simulink model "WS1Sol"  (R2019b)
settings: Solver=VariableStepAuto  StartTime=0.0  StopTime=10  RelTol=1e-3
libraries: dspsrcs4 x2, simulink_extras x1
settings Model: Creator=Shishir  LastModifiedBy=Shishir

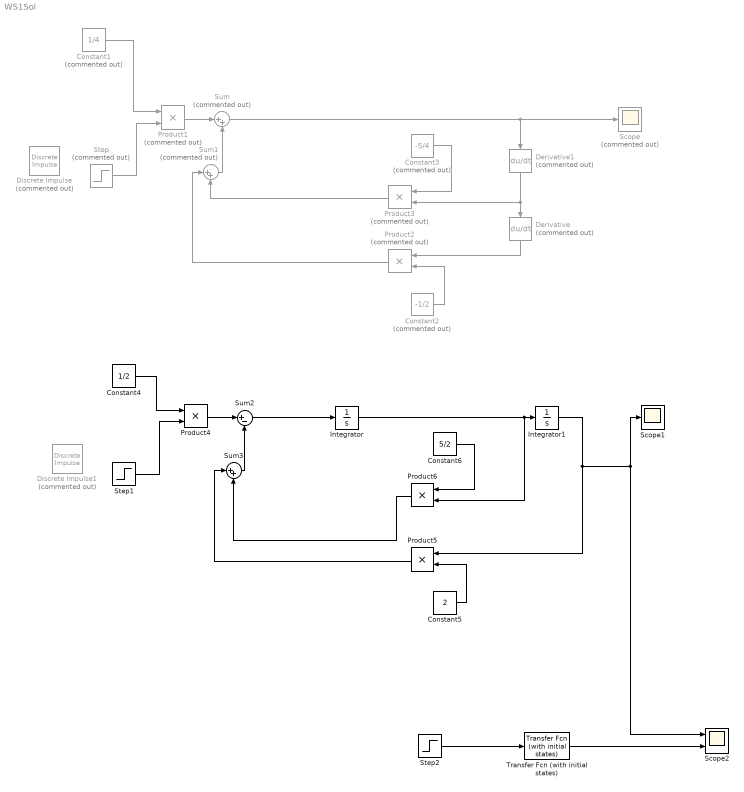
== system WS1Sol ==
  Constant1 : Constant  Commented=on  Value=1/4
  Constant2 : Constant  Commented=on  Value=-1/2
  Constant3 : Constant  Commented=on  Value=-5/4
  Constant4 : Constant  Value=1/2
  Constant5 : Constant  Value=2
  Constant6 : Constant  Value=5/2
  Derivative : Derivative  Commented=on
  Derivative1 : Derivative  Commented=on
  Discrete Impulse : dspsrcs4/Discrete  Impulse  Commented=on  Delay=0  SampleTime=1  FrameSample=1  OutputFrames=off  dataType=double  isSigned=on  wordLen=16  udDataType=sfix(16)  fracBitsMode=Best precision  numFracBits=15  OutDataTypeStr=double  LastOutDataTypeStr=double
  Discrete Impulse1 : dspsrcs4/Discrete  Impulse  Commented=on  Delay=0  SampleTime=1  FrameSample=1  OutputFrames=off  dataType=double  isSigned=on  wordLen=16  udDataType=sfix(16)  fracBitsMode=Best precision  numFracBits=15  OutDataTypeStr=double  LastOutDataTypeStr=double
  Integrator : Integrator
  Integrator1 : Integrator
  Product1 : Product  Commented=on
  Product2 : Product  Commented=on
  Product3 : Product  Commented=on
  Product4 : Product
  Product5 : Product
  Product6 : Product
  Scope : Scope  Commented=on
  Scope1 : Scope
  Scope2 : Scope  NumInputPorts=2
  Step : Step  Commented=on  SampleTime=0
  Step1 : Step  SampleTime=0
  Step2 : Step  SampleTime=0
  Sum : Sum  Commented=on  Inputs=|++
  Sum1 : Sum  Commented=on  Inputs=|++
  Sum2 : Sum  Inputs=|+-
  Sum3 : Sum  Inputs=|++
  Transfer Fcn (with initial states) : simulink_extras/Additional Linear/Transfer Fcn (with initial states)  N=[1]  D="[2  5 4]"  X0=0
  wires:
  Product1/1 -> Sum/1
  Step/1 -> Product1/2
  Constant1/1 -> Product1/1
  Sum/1 -> Derivative1/1, Scope/1
  Derivative1/1 -> Product3/2, Derivative/1
  Sum1/1 -> Sum/2
  Product3/1 -> Sum1/2
  Product2/1 -> Sum1/1
  Constant3/1 -> Product3/1
  Constant2/1 -> Product2/2
  Derivative/1 -> Product2/1
  Product4/1 -> Sum2/1
  Step1/1 -> Product4/2
  Integrator1/1 -> Product5/1, Scope2/1, Scope1/1
  Constant6/1 -> Product6/1
  Product6/1 -> Sum3/2
  Constant4/1 -> Product4/1
  Constant5/1 -> Product5/2
  Product5/1 -> Sum3/1
  Sum3/1 -> Sum2/2
  Integrator/1 -> Product6/2, Integrator1/1
  Sum2/1 -> Integrator/1
  Step2/1 -> Transfer Fcn (with initial states)/1
  Transfer Fcn (with initial states)/1 -> Scope2/2
